simulink subsystem "DM_SystemDiagnostics"  (R2019b)
settings: Solver=VariableStepAuto  StartTime=0.0  StopTime=10.0  RelTol=1e-3
libraries: FaultDetector x1
settings Model: Creator=Nick  LastModifiedBy=Nick

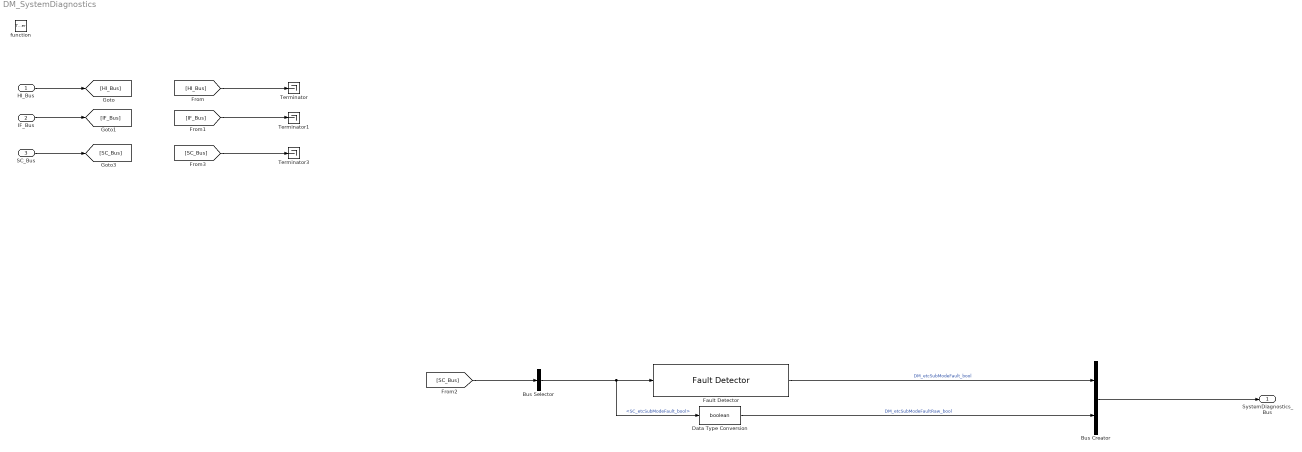
== system DM_SystemDiagnostics ==
  HI_Bus : Inport
  IF_Bus : Inport  Port=2
  SC_Bus : Inport  Port=3
  function : TriggerPort  TriggerType=function-call  VariantControl=Variant
  Bus Creator : BusCreator  Inputs=2
  Bus Selector : BusSelector  OutputSignals=modeControlBus.SC_etcSubModeFault_bool
  Data Type Conversion : DataTypeConversion  OutDataTypeStr=boolean
  Fault Detector : FaultDetector/Fault Detector  timeTrip=1  timeReset=1  isSticky=off
  Terminator : Terminator
  Terminator1 : Terminator
  Terminator3 : Terminator
  SystemDiagnostics_Bus : Outport
  wires:
  Data Type Conversion/1 -> Bus Creator/2  "DM_etcSubModeFaultRaw_bool"
  Fault Detector/1 -> Bus Creator/1  "DM_etcSubModeFault_bool"
  Bus Selector/1 -> Data Type Conversion/1, Fault Detector/1  "<SC_etcSubModeFault_bool>"
  [SC_Bus] -> Bus Selector/1
  Bus Creator/1 -> SystemDiagnostics_Bus/1
  SC_Bus/1 -> [SC_Bus]
  [SC_Bus] -> Terminator3/1
  HI_Bus/1 -> [HI_Bus]
  IF_Bus/1 -> [IF_Bus]
  [HI_Bus] -> Terminator/1
  [IF_Bus] -> Terminator1/1
